simulink model "clase2"  (Simulink 7.9)
settings: Solver=ode45  StartTime=0.0  StopTime=10.0  RelTol=1e-3
settings Model: Creator=diegodorado  LastModifiedBy=diegodorado

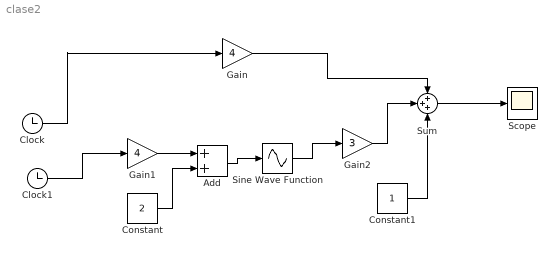
== system clase2 ==
  Add : Sum
  Clock : Clock
  Clock1 : Clock
  Constant : Constant  Value=2
  Constant1 : Constant
  Gain : Gain  Gain=4
  Gain1 : Gain  Gain=4
  Gain2 : Gain  Gain=3
  Scope : Scope
  Sine Wave Function : Sin  TimeSource=Use external signal  SampleTime=0
  Sum : Sum  Inputs=+++
  wires:
  Sum/1 -> Scope/1
  Clock/1 -> Gain/1
  Gain/1 -> Sum/1
  Constant1/1 -> Sum/3
  Sine Wave Function/1 -> Gain2/1
  Gain2/1 -> Sum/2
  Gain1/1 -> Add/1
  Add/1 -> Sine Wave Function/1
  Constant/1 -> Add/2
  Clock1/1 -> Gain1/1
